simulink model "roll_sim"  (Simulink 8.1)
settings: Solver=FixedStepDiscrete  SolverMode=SingleTasking  StartTime=0.0  StopTime=10.0  RelTol=1e-3
libraries: sphero_lib x3
settings Model: Creator=gcampa  LastModifiedBy=gcampa
settings DataIOCC: SignalLoggingSaveFormat=Dataset
settings OptimizationCC: BlockReduction=off  BooleanDataType=off  ExpressionDepthLimit=128
settings DebuggingCC: SaveWithParameterizedLinksMsg=none  SignalResolutionControl=TryResolveAllWithWarning  SolverPrmCheckMsg=none  FcnCallInpInsideContextMsg=EnableAllAsError  StateNameClashWarn=none
settings HardwareCC: TargetUnknown=on
settings GRTTargetCC: CodeReplacementLibrary=C89/C90 (ANSI)  CombineOutputUpdateFcns=on  GRTInterface=off

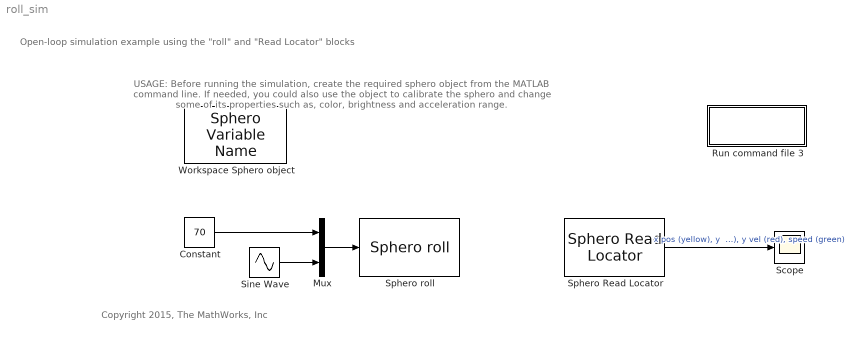
== system roll_sim ==
  note: Open-loop simulation example using the "roll" and "Read Locator" blocks
  note: Copyright 2015, The MathWorks, Inc
  note: USAGE:
      | Before running the simulation, create the required sphero object
      | from the MATLAB command line. If needed, you could also use
      | the object to calibrate the sphero and change some of its properties
      | such as, color, brightness and acceleration range.
  Constant : Constant  Value=70
  Mux : Mux  Inputs=2
  Run command file 3 : Subsystem
      settings: OpenFcn=sphero_lib
      mask Display: disp('Open Main\nSimulink Library')
  Scope : Scope
      settings: TimeRange=10  YMin=-1000  YMax=1000  SaveName=yout
  Sine Wave : Sin  Amplitude=360  Frequency=pi/2/5  SampleTime=0.2
  Sphero Read Locator : sphero_lib/Sphero Read Locator  SpheroVarNumber=Existing workspace Sphero variable #1  T=0.2
  Sphero roll : sphero_lib/Sphero roll  SpheroVarNumber=Existing workspace Sphero variable #1  T=0.2
  Workspace Sphero object : sphero_lib/Sphero Variable Name  Priority=3  SpheroVarNumber=Existing workspace Sphero variable #1  workspaceVarName=sph
  wires:
  Sphero Read Locator/1 -> Scope/1  "x pos (yellow), y  pos (magenta), x vel (cyan), y vel (red), speed (green)"
  Mux/1 -> Sphero roll/1
  Constant/1 -> Mux/1
  Sine Wave/1 -> Mux/2

== system roll_sim/Run command file 3 ==
